simulink model "sFlow_Raul_V3"  (R2017a)
settings: Solver=VariableStepAuto  StartTime=0.0  StopTime=1  MaxStep=1e-6  RelTol=1e-3
libraries: simulink_extras x2, mpclib x1, powerlib_meascontrol x1
settings Model: Creator=erich  LastModifiedBy=erich
settings SolverCC: ZeroCrossAlgorithm=Adaptive

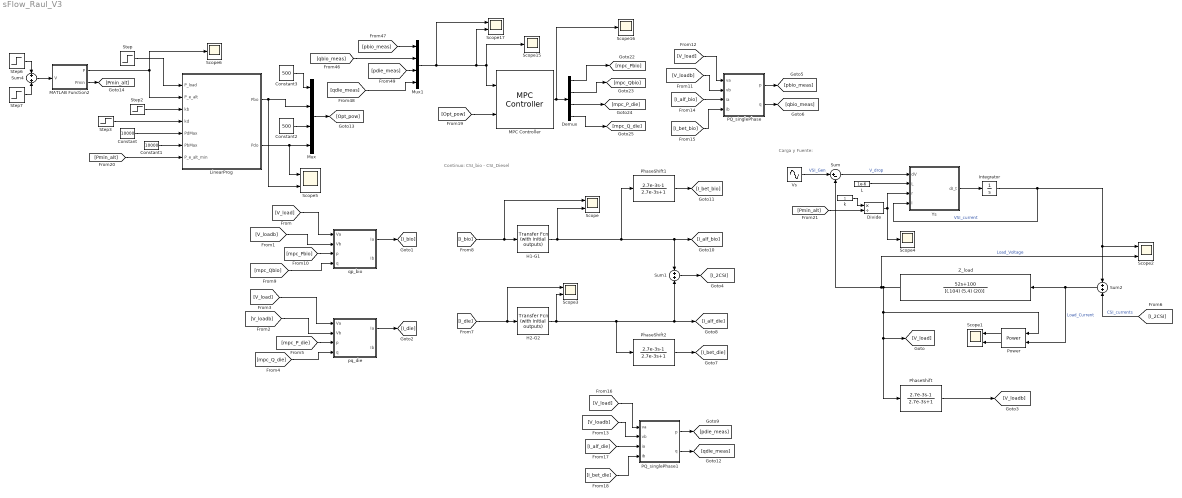
== system sFlow_Raul_V3 ==
  note: Continuo: CSI_bio - CSI_Diesel
  note: Carga y Fuente:
  Constant : Constant  Value=10000
  Constant1 : Constant  Value=10000
  Constant2 : Constant  Value=500
  Constant3 : Constant  Value=500
  Demux : Demux
  Divide : Product  Inputs=*/
  H1-G1 : simulink_extras/Additional Linear/Transfer Fcn (with initial outputs)  N="[0 0 6726810176.12524 6.73124120936324e+15 6.50924655818422e+19 4.05177167314893e+23 3.22856603808296e+27\t3.14408741016115e+30 1.65038796373999e+33 4.40591526133565e+35 6.17957736022027e+37 1.17231652164067e+38]"  D=[1 2000160.68008932 1016066493843.91 1.59653892356830e+16 1.20684541605981e+20 8.53045931700448e+23 3.46928633693524e+27 3.27211364208147e+30 1.68376309840209e+33 4.49704200624656e+35 6.18358109583087e+37 1.17275182947158e+38]  Y0=0  U0=0
  H2-G2 : simulink_extras/Additional Linear/Transfer Fcn (with initial outputs)  N="[0 0 8969080234.83366 8.97498080491745e+15 6.66737187257785e+19 5.16949832616537e+23 3.28496501858301e+27\t3.17590820302043e+30 1.65840204844398e+33 4.42846963810343e+35 6.18000819896227e+37 1.17231652164089e+38]"  D=[1 2000160.68008932 1016066493843.91 1.59653892356830e+16 1.20684541605981e+20 8.53045931700448e+23 3.46928633693524e+27 3.27211364208147e+30 1.68376309840209e+33 4.49704200624656e+35 6.18358109583087e+37 1.17275182947158e+38]  Y0=0  U0=0
  Integrator : Integrator
  L : Constant  Value=1e-6
  LinearProg : MATLAB Function  TreatAsAtomicUnit=on
  MATLAB Function2 : MATLAB Function  TreatAsAtomicUnit=on
  MPC Controller : mpclib/MPC Controller  SCDEnableBlockLinearizationSpecification=on  mpcobj=mpcobj  is_multiple=0  enable_value=0  return_u0=off  ref_from_ws=off  ref_signal_name=[]  ref_preview=off  md_from_ws=off  md_signal_name=[]  md_preview=off  from_project=off  project_file=MPCtask.mat  md_inport=off  mv_inport=off  cost_outport=off  return_sequence=off  return_qpstatus=off  return_state=off  state_inport=off  lims_inport=off  ywt_inport=off  is_designfromscratch=0  uwt_inport=off  duwt_inport=off  rhoeps_inport=off  uref_inport=off  n_ts=0.03  n_mv=4  n_md=0  n_ud=0  n_mo=4  n_uo=0  BlockDataType=double  SampleTimeInherited=off  switch_inport=off
  Mux : Mux
  Mux1 : Mux
  PQ_singlePhase : MATLAB Function  TreatAsAtomicUnit=on
  PQ_singlePhase1 : MATLAB Function  TreatAsAtomicUnit=on
  PhaseShift : TransferFcn  Numerator=[2.7e-3 -1]  Denominator=[2.7e-3 1]
  PhaseShift1 : TransferFcn  Numerator=[2.7e-3 -1]  Denominator=[2.7e-3 1]
  PhaseShift2 : TransferFcn  Numerator=[2.7e-3 -1]  Denominator=[2.7e-3 1]
  Power : powerlib_meascontrol/Measurements/Power  Freq=60  Vinit=[1, 0]  Iinit=[1, 0]  Ts=0
      settings: SourceProductName=Simscape Power Systems
  Scope{,1..3,5,17} (6 alike) : Scope  NumInputPorts=2
  Scope{4,6,15..16} (4 alike) : Scope
  Step : Step  Time=.2  Before=5000  After=10000  SampleTime=0
  Step2 : Step  Time=.2  Before=1.2  After=1.2  SampleTime=0
  Step3 : Step  Time=.2  Before=.7  After=.7  SampleTime=0
  Step6 : Step  Time=.2  Before=12  After=22  SampleTime=0
  Step7 : Step  Time=.5  After=-17  SampleTime=0
  Sum : Sum  Inputs=|+-
  Sum1 : Sum  Inputs=+|+
  Sum2 : Sum  Inputs=+|+
  Sum4 : Sum  Inputs=+|+
  Vs : Sin  Amplitude=170  Frequency=2*pi*60  SampleTime=0
  Ys : MATLAB Function  TreatAsAtomicUnit=on
  Z_load : TransferFcn  Numerator=[52 100]  Denominator=[(.104) (5.4) (20)]
  k : Constant
  pq_die : MATLAB Function  TreatAsAtomicUnit=on
  qp_bio : MATLAB Function  TreatAsAtomicUnit=on
  wires:
  [I_bio] -> Scope/1, H1-G1/1
  H1-G1/1 -> PhaseShift1/1, [I_alf_bio], Sum1/1, Scope/2
  H2-G2/1 -> Scope3/2, [I_alf_die], Sum1/2, PhaseShift2/1
  [I_die] -> Scope3/1, H2-G2/1
  qp_bio/1(Ia) -> [I_bio]
  pq_die/1(Ia) -> [I_die]
  Sum1/1 -> [I_2CSI]
  PhaseShift/1 -> [V_loadb]
  [V_loadb] -> pq_die/2(Vb)
  [V_load] -> pq_die/1(Va)
  [V_loadb] -> qp_bio/2(Vb)
  [V_load] -> qp_bio/1(Va)
  Mux1/1 -> Scope17/2, MPC Controller/1, Scope15/1, Scope17/1
  [pbio_meas] -> Mux1/1
  [Opt_pow] -> MPC Controller/2
  [pdie_meas] -> Mux1/3
  [qbio_meas] -> Mux1/2
  Demux/2 -> [mpc_Qbio]
  Demux/1 -> [mpc_Pbio]
  MPC Controller/1 -> Scope16/1, Demux/1
  Demux/3 -> [mpc_P_die]
  Demux/4 -> [mpc_Q_die]
  [qdie_meas] -> Mux1/4
  [mpc_Pbio] -> qp_bio/3(p)
  [mpc_Qbio] -> qp_bio/4(q)
  [mpc_P_die] -> pq_die/3(p)
  [mpc_Q_die] -> pq_die/4(q)
  [V_load] -> PQ_singlePhase/1(va)
  [V_loadb] -> PQ_singlePhase/2(vb)
  [I_bet_bio] -> PQ_singlePhase/4(ib)
  [I_alf_bio] -> PQ_singlePhase/3(ia)
  PQ_singlePhase/1(p) -> [pbio_meas]
  PQ_singlePhase/2(q) -> [qbio_meas]
  PhaseShift1/1 -> [I_bet_bio]
  PhaseShift2/1 -> [I_bet_die]
  [I_alf_die] -> PQ_singlePhase1/3(ia)
  [I_bet_die] -> PQ_singlePhase1/4(ib)
  PQ_singlePhase1/2(q) -> [qdie_meas]
  [V_load] -> PQ_singlePhase1/1(va)
  PQ_singlePhase1/1(p) -> [pdie_meas]
  [V_loadb] -> PQ_singlePhase1/2(vb)
  Step/1 -> LinearProg/1(P_load)
  MATLAB Function2/1(P) -> Scope6/1, LinearProg/2(P_e_alt)
  Constant/1 -> LinearProg/5(PdMax)
  Constant1/1 -> LinearProg/6(PbMax)
  Step2/1 -> LinearProg/3(kb)
  Step3/1 -> LinearProg/4(kd)
  LinearProg/2(Pdo) -> Scope5/1, Mux/4
  LinearProg/1(Pbo) -> Scope5/2, Mux/2
  Mux/1 -> [Opt_pow]
  Constant2/1 -> Mux/3
  Constant3/1 -> Mux/1
  [I_2CSI] -> Sum2/2  "CSI_currents"
  Sum2/1 -> Power/2, Z_load/1  "Load_Current"
  Z_load/1 -> PhaseShift/1, [V_load], Power/1, Scope2/2, Sum/2  "Load_Voltage"
  Power/1 -> Scope1/1
  Power/2 -> Scope1/2
  Vs/1 -> Sum/1  "VSI_Gen"
  Sum/1 -> Ys/1(dV)  "V_drop"
  L/1 -> Ys/2(L)
  Ys/1(dI_t) -> Integrator/1
  Integrator/1 -> Scope2/1, Sum2/1, Ys/4(I)  "VSI_current"
  Step7/1 -> Sum4/2
  Sum4/1 -> MATLAB Function2/1(V)
  Step6/1 -> Sum4/1
  MATLAB Function2/2(Pmin) -> [Pmin_alt]
  [Pmin_alt] -> LinearProg/7(P_e_alt_min)
  [Pmin_alt] -> Divide/2
  k/1 -> Divide/1
  Divide/1 -> Scope4/1, Ys/3(r)

== matlab function sFlow_Raul_V3/pq_die ==
  data: Va input; Ia output; Vb input; p input; q input; Ib output
function [Ia, Ib] = fcn(Va, Vb, p, q)
%#codegen

% divide by zero protection
if(abs((Va^2+Vb^2))<=1000*eps(0))
    det = 1/eps(0);
else
    det = 1/(Va^2+Vb^2); % constante auxiliar
end;
%det = 1/(Va^2+Vb^2);

Mat = det*[Va Vb; Vb -Va];
Iab = Mat*[2*p;2*q];

Iaaux = Iab(1);
Ibaux = Iab(2);

ilim=1e3;

if(Iaaux>ilim)
    Iaaux=ilim;
end;
if(Iaaux<-ilim)
    Iaaux =-ilim;    
end;

if(isnan(Iaaux))
    Iaaux=0;
end;
%-----------------


if(Ibaux>ilim)
    Ibaux=ilim;
end;
if(Ibaux<-ilim)
    Ibaux =-ilim;    
end;

if(isnan(Ibaux))
    Ibaux=0;
end;
%-----------------


Ia = Iaaux;
Ib = Ibaux;

== matlab function sFlow_Raul_V3/PQ_singlePhase1 ==
  data: va input; p output; vb input; ia input; ib input; q output
function [p, q] = fcn(va, vb, ia, ib)
% Esta funcion calcula la potencia activa y reactiva instantanea
% para el caso mnosofasico. En la revision de 2 papers he observado
% que una manera de extender la teoria de potencia al caso monofasico
% es asumiendo la tension o corriente de una fase como la componente
% alpha y hacer un desfase de 90 grados para obtener una version
% artificial de beta.

paux=va*ia+vb*ib;
if(paux > 20e4)
    paux = 20e4;
end
if(paux < -20e4)
    paux = -20e-4;
end

p = paux/2; % potencia activa instantanea

qaux = vb*ia-va*ib;

if(qaux>20e4)
    qaux=20e4;
end
if(qaux<-20e4)
    qaux=-20e4;
end

q = qaux/2; % potencia reactiva instantanea

== matlab function sFlow_Raul_V3/PQ_singlePhase ==
  data: va input; p output; vb input; ia input; ib input; q output
function [p, q] = fcn(va, vb, ia, ib)
% Esta funcion calcula la potencia activa y reactiva instantanea
% para el caso mnosofasico. En la revision de 2 papers he observado
% que una manera de extender la teoria de potencia al caso monofasico
% es asumiendo la tension o corriente de una fase como la componente
% alpha y hacer un desfase de 90 grados para obtener una version
% artificial de beta.

paux=va*ia+vb*ib;
if(paux > 20e4)
    paux = 20e4;
end
if(paux < -20e4)
    paux = -20e-4;
end

p = paux/2; % potencia activa instantanea

qaux = vb*ia-va*ib;

if(qaux>20e4)
    qaux=20e4;
end
if(qaux<-20e4)
    qaux=-20e4;
end

q = qaux/2; % potencia reactiva instantanea

== matlab function sFlow_Raul_V3/LinearProg ==
  data: P_load input; Pbo output; P_e_alt input; kb input; kd input; PdMax input; PbMax input; Pdo output; P_e_alt_min input
function [Pbo, Pdo] = fcn(P_load, P_e_alt, kb, kd, PdMax, PbMax, P_e_alt_min)

% P_load es la potencia que se requiere en la carga.

% P_e_alt es la potencia estimada de generacion de las energias
% alternativas

% kb y kd son los pesos de las funcion de costo.

% las salidas son las potencias optimas para bio y diesel

Pb=0;
Pd=0;

D_P_e_alt = P_e_alt - P_e_alt_min % superaavit de energia alternativa.

flagDelt = 0;

if(D_P_e_alt >= P_load)
    flagDelt = 1;
end
   

if(flagDelt==0)
    P_trad = P_load - D_P_e_alt;
    % flag: variable que indica si tiene sentido evaluar los
    % if's que se encuentran mas adelante. es decir, si flag = 0 
    % despues del primer if entonces NO se le esta pidiendo al sistema
    % mas potencia de la que puede generar y portante el problema de 
    % optimizacion lineal tiene sentido.
    % entonces 
    flag=0;

    if(P_trad>PdMax+PbMax)
        Pd=PdMax;
        Pb=PbMax;
        flag=1;
    end

    % si ambas energias tienen el mismo factor de costo.
    if(kd==kb && flag==0)
        Pb=P_trad/2;
        Pd=P_trad/2;
    end

    % si la energia diesel es mas cara que la biomasa.
    if(kd>kb && flag==0)
        if(P_trad<=PbMax)
            Pb=P_trad;
            Pd=0;
        else
            Pb=PbMax;
            Pd=P_trad-PbMax;
        end
    end

    % si la biomasa es mas cara que la diesel.
    if(kd<kb && flag==0)
        if(P_trad<=PdMax)
            Pd=P_trad;
            Pb=0;
        else
            Pd=PdMax;
            Pb=P_trad-PdMax;
        end
    end
end

Pbo=Pb;
Pdo=Pd;

== matlab function sFlow_Raul_V3/Ys ==
  data: dV input; dI_t output; L input; r input; I input
function dI_t = fcn(dV, L, r, I)

dI_t = dV/L - I*r/(L);

== matlab function sFlow_Raul_V3/MATLAB Function2 ==
  data: V input; P output; Pmin output
function [P, Pmin]= fcn(V)

P=0;
m=0;
b=0;

vfull = 16;
vexp = 14;
vnom = 8;

m1 = 11000/12;
m2 = 1000/(vexp-vnom);
m3 = 10*(1000/(vexp-vnom));

b1 = 0;
b2 = m1*vnom-m2*vnom;
b3 = m2*vexp+b2-m3*vexp;

if(V>=0 && V<vnom)
    m=m1;
    b=b1;
end

if(V>=vnom && V<vexp)
    m=m2;
    b=b2;
end

if(V>=vexp)
    m=m3;
    b=b3;
end

P=m*V + b;

if(V<0)
    P=0;
end

Pmin=m1*vnom;

== matlab function sFlow_Raul_V3/qp_bio ==
  data: Va input; Ia output; Vb input; p input; q input; Ib output
function [Ia, Ib] = fcn(Va, Vb, p, q)
%#codegen

% divide by zero protection
if(abs((Va^2+Vb^2))<=1000*eps(0))
    det = 1/eps(0);
else
    det = 1/(Va^2+Vb^2); % constante auxiliar
end;
%det = 1/(Va^2+Vb^2);

Mat = det*[Va Vb; Vb -Va];
Iab = Mat*[2*p;2*q];

Iaaux = Iab(1);
Ibaux = Iab(2);

ilim=1e3;

if(Iaaux>ilim)
    Iaaux=ilim;
end;
if(Iaaux<-ilim)
    Iaaux =-ilim;    
end;

if(isnan(Iaaux))
    Iaaux=0;
end;
%-----------------


if(Ibaux>ilim)
    Ibaux=ilim;
end;
if(Ibaux<-ilim)
    Ibaux =-ilim;    
end;

if(isnan(Ibaux))
    Ibaux=0;
end;
%-----------------


Ia = Iaaux;
Ib = Ibaux;
